simulink model "majority_3bit"  (R2025b)
settings: Solver=VariableStepAuto  StartTime=0.0  StopTime=10.0  RelTol=1e-3
settings Model: Creator=Johan  LastModifiedBy=Johan

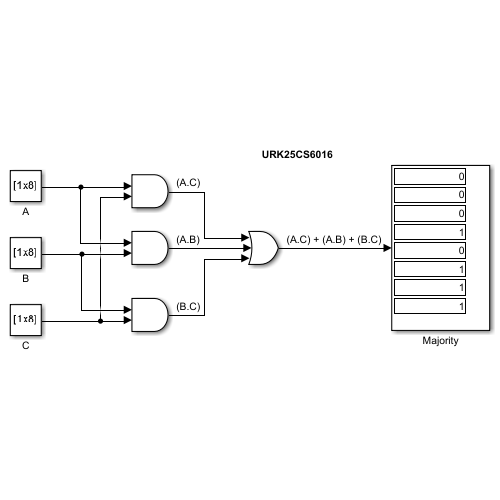
[thumbnail: Simulink's stored preview of the top-level diagram]
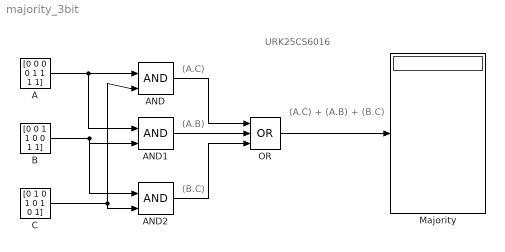
== system majority_3bit ==
  note: URK25CS6016
  note: (A.C)
  note: (A.B)
  note: (B.C)
  note: (A.C) + (A.B) + (B.C)
  A : Constant  Value=[0 0 0 0 1 1 1 1]
  AND : Logic  IconShape=distinctive  AllPortsSameDT=off  OutDataTypeStr=boolean
  AND1 : Logic  IconShape=distinctive  AllPortsSameDT=off  OutDataTypeStr=boolean
  AND2 : Logic  IconShape=distinctive  AllPortsSameDT=off  OutDataTypeStr=boolean
  B : Constant  Value=[0 0 1 1 0 0 1 1]
  C : Constant  Value=[0 1 0 1 0 1 0 1]
  Majority : Display
  OR : Logic  Operator=OR  Inputs=3  IconShape=distinctive  AllPortsSameDT=off  OutDataTypeStr=boolean
  wires:
  A/1 -> AND1/1, AND/1
  C/1 -> AND/2, AND2/2
  B/1 -> AND2/1, AND1/2
  AND/1 -> OR/1
  AND1/1 -> OR/2
  AND2/1 -> OR/3
  OR/1 -> Majority/1
